simulink library "CTRL_LO_ST1_DFLATLGT"  (R2023b)
settings: Solver=VariableStepAuto  StartTime=0.0  StopTime=10.0  RelTol=1e-3
undefined symbols (not defined in the file): CTRL_LO_ST1_p_DeltaFLgt_N
settings Model: Creator=blatak  LastModifiedBy=blatak

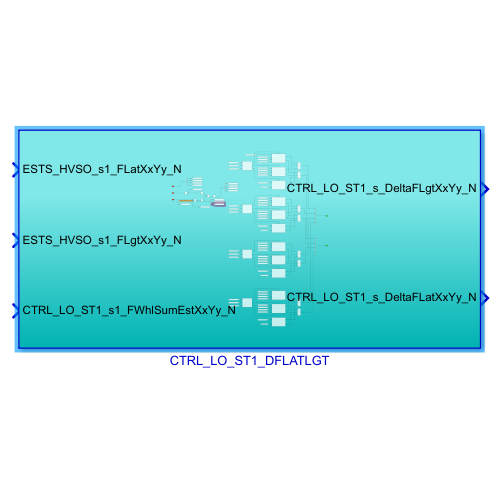
[thumbnail: Simulink's stored preview of the top-level diagram]
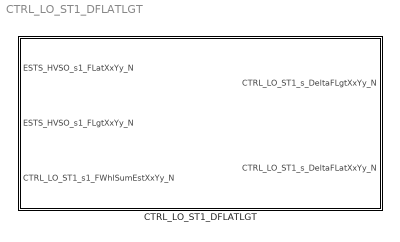
== system CTRL_LO_ST1_DFLATLGT ==
  CTRL_LO_ST1_DFLATLGT : Subsystem

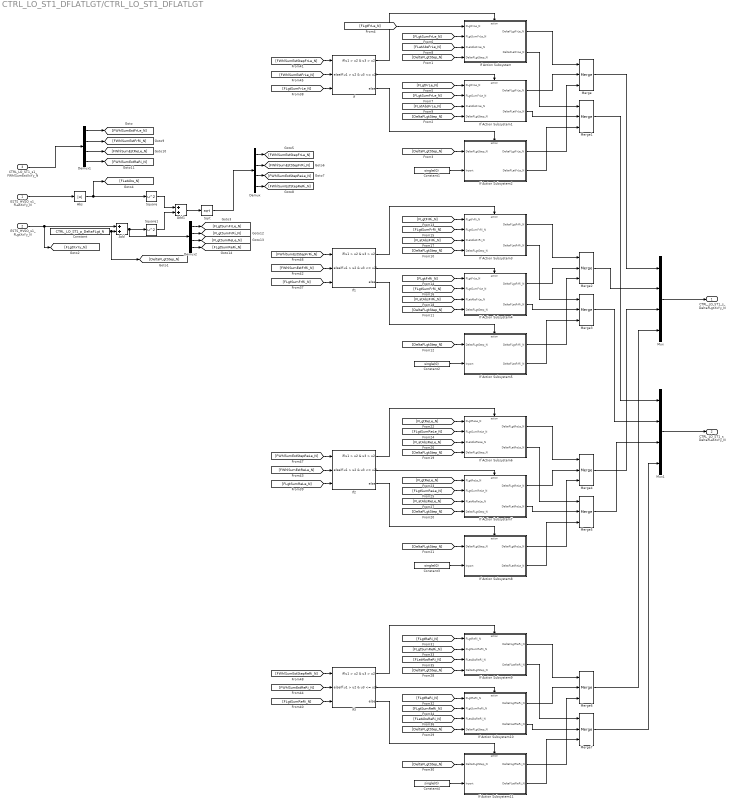
== system CTRL_LO_ST1_DFLATLGT/CTRL_LO_ST1_DFLATLGT ==
  ESTS_HVSO_s1_FLatXxYy_N : Inport
  ESTS_HVSO_s1_FLgtXxYy_N : Inport  Port=2
  CTRL_LO_ST1_s1_FWhlSumEstXxYy_N : Inport  Port=3
  Abs : Abs  SaturateOnIntegerOverflow=off
  Add : Sum
  Add1 : Sum
  Constant : Constant  Value=CTRL_LO_ST1_p_DeltaFLgt_N
  Constant{1..4} (4 alike) : Constant  Value=single(0)
  Demux : Demux
  Demux1 : Demux
  Demux2 : Demux
  If{,1..3} (4 alike) : If  NumInputs=3  IfExpression=u1 > u2 & u3 > u2  ElseIfExpressions=u1 > u2 & u3 <= u2
  If Action Subsystem : Subsystem  TreatAsAtomicUnit=on
  If Action Subsystem1 : Subsystem  TreatAsAtomicUnit=on
  If Action Subsystem10 : Subsystem  AncestorBlock=CTRL_LO_ST1_DFLATLGT/CTRL_LO_ST1_DFLATLGT/If Action Subsystem1  TreatAsAtomicUnit=on
  If Action Subsystem11 : Subsystem  AncestorBlock=CTRL_LO_ST1_DFLATLGT/CTRL_LO_ST1_DFLATLGT/If Action Subsystem2  TreatAsAtomicUnit=on
  If Action Subsystem2 : Subsystem  TreatAsAtomicUnit=on
  If Action Subsystem3 : Subsystem  AncestorBlock=CTRL_LO_ST1_DFLATLGT/CTRL_LO_ST1_DFLATLGT/If Action Subsystem  TreatAsAtomicUnit=on
  If Action Subsystem4 : Subsystem  AncestorBlock=CTRL_LO_ST1_DFLATLGT/CTRL_LO_ST1_DFLATLGT/If Action Subsystem1  TreatAsAtomicUnit=on
  If Action Subsystem5 : Subsystem  AncestorBlock=CTRL_LO_ST1_DFLATLGT/CTRL_LO_ST1_DFLATLGT/If Action Subsystem2  TreatAsAtomicUnit=on
  If Action Subsystem6 : Subsystem  AncestorBlock=CTRL_LO_ST1_DFLATLGT/CTRL_LO_ST1_DFLATLGT/If Action Subsystem  TreatAsAtomicUnit=on
  If Action Subsystem7 : Subsystem  AncestorBlock=CTRL_LO_ST1_DFLATLGT/CTRL_LO_ST1_DFLATLGT/If Action Subsystem1  TreatAsAtomicUnit=on
  If Action Subsystem8 : Subsystem  AncestorBlock=CTRL_LO_ST1_DFLATLGT/CTRL_LO_ST1_DFLATLGT/If Action Subsystem2  TreatAsAtomicUnit=on
  If Action Subsystem9 : Subsystem  AncestorBlock=CTRL_LO_ST1_DFLATLGT/CTRL_LO_ST1_DFLATLGT/If Action Subsystem  TreatAsAtomicUnit=on
  Merge{,1..7} (8 alike) : Merge  Inputs=3
  Mux : Mux
  Mux1 : Mux
  Sqrt : Sqrt
  Square : Math  Operator=square
  Square1 : Math  Operator=square
  CTRL_LO_ST1_s_DeltaFLgtXxYy_N : Outport
  CTRL_LO_ST1_s_DeltaFLatXxYy_N : Outport  Port=2
  wires:
  Abs/1 -> [FLatAbs_N], Square/1
  Add1/1 -> Sqrt/1
  Square/1 -> Add1/1
  Add/1 -> Demux2/1, Square1/1
  If Action Subsystem/1(DeltaFLgtFrLe_N) -> Merge/1
  Merge/1 -> Mux/1
  If/2 -> If Action Subsystem1/Action
  If Action Subsystem2/1(DeltaFLgtFrLe_N) -> Merge/3
  Constant/1 -> [DeltaFLgtStep_N], Add/2
  [FLgtSumFrLe_N] -> If Action Subsystem1/2(FLgtSumFrLe_N)
  If Action Subsystem2/2(DeltaFLatFrLe_N) -> Merge1/3
  [DeltaFLgtStep_N] -> If Action Subsystem2/1(DeltaFLgtStep_N)
  ESTS_HVSO_s1_FLgtXxYy_N/1 -> [FLgtXxYy_N], Add/1
  If Action Subsystem1/2(DeltaFLatFrLe_N) -> Merge1/2
  Sqrt/1 -> Demux/1
  [FLgtSumFrLe_N] -> If Action Subsystem/2(FLgtSumFrLe_N)
  [FLgtFrLe_N] -> If Action Subsystem1/1(FLgtFrLe_N)
  [FLatAbsFrLe_N] -> If Action Subsystem1/3(FLatAbsFrLe_N)
  [DeltaFLgtStep_N] -> If Action Subsystem/4(DeltaFLgtStep_N)
  Square1/1 -> Add1/2
  [DeltaFLgtStep_N] -> If Action Subsystem1/4(DeltaFLgtStep_N)
  Constant1/1 -> If Action Subsystem2/2(Inport)
  ESTS_HVSO_s1_FLatXxYy_N/1 -> Abs/1
  CTRL_LO_ST1_s1_FWhlSumEstXxYy_N/1 -> Demux1/1
  Merge1/1 -> Mux1/1
  [FLgtFrLe_N] -> If Action Subsystem/1(FLgtFrLe_N)
  If/3 -> If Action Subsystem2/Action
  [FLatAbsFrLe_N] -> If Action Subsystem/3(FLatAbsFrLe_N)
  If Action Subsystem1/1(DeltaFLgtFrLe_N) -> Merge/2
  If/1 -> If Action Subsystem/Action
  If Action Subsystem/2(DeltaFLatFrLe_N) -> Merge1/1
  If Action Subsystem5/2(DeltaFLatFrRi_N) -> Merge3/3
  Merge2/1 -> Mux/2
  [FLatAbsFrRi_N] -> If Action Subsystem4/3(FLatAbsFrLe_N)
  If Action Subsystem4/2(DeltaFLatFrRi_N) -> Merge3/2
  [FLgtSumFrRi_N] -> If Action Subsystem3/2(FLgtSumFrRi_N)
  [FLgtFrRi_N] -> If Action Subsystem4/1(FLgtFrLe_N)
  If Action Subsystem3/2(DeltaFLatFrRi_N) -> Merge3/1
  If Action Subsystem4/1(DeltaFLgtFrRi_N) -> Merge2/2
  If1/1 -> If Action Subsystem3/Action
  [DeltaFLgtStep_N] -> If Action Subsystem4/4(DeltaFLgtStep_N)
  [FLgtFrRi_N] -> If Action Subsystem3/1(FLgtFrRi_N)
  Constant2/1 -> If Action Subsystem5/2(Inport)
  [FLatAbsFrRi_N] -> If Action Subsystem3/3(FLatAbsFrRi_N)
  If1/3 -> If Action Subsystem5/Action
  If1/2 -> If Action Subsystem4/Action
  [FLgtSumFrRi_N] -> If Action Subsystem4/2(FLgtSumFrLe_N)
  [DeltaFLgtStep_N] -> If Action Subsystem5/1(DeltaFLgtStep_N)
  [DeltaFLgtStep_N] -> If Action Subsystem3/4(DeltaFLgtStep_N)
  If Action Subsystem3/1(DeltaFLgtFrRi_N) -> Merge2/1
  If Action Subsystem5/1(DeltaFLgtFrRi_N) -> Merge2/3
  Merge3/1 -> Mux1/2
  If Action Subsystem8/2(DeltaFLatReLe_N) -> Merge5/3
  Merge4/1 -> Mux/3
  [FLatAbsReLe_N] -> If Action Subsystem7/3(FLatAbsReLe_N)
  If Action Subsystem7/2(DeltaFLatReLe_N) -> Merge5/2
  [FLgtSumReLe_N] -> If Action Subsystem6/2(FLgtSumReLe_N)
  [FLgtReLe_N] -> If Action Subsystem7/1(FLgtReLe_N)
  If Action Subsystem6/2(DeltaFLatReLe_N) -> Merge5/1
  If Action Subsystem7/1(DeltaFLgtReLe_N) -> Merge4/2
  If2/1 -> If Action Subsystem6/Action
  [DeltaFLgtStep_N] -> If Action Subsystem7/4(DeltaFLgtStep_N)
  [FLgtReLe_N] -> If Action Subsystem6/1(FLgtReLe_N)
  Constant3/1 -> If Action Subsystem8/2(Inport)
  [FLatAbsReLe_N] -> If Action Subsystem6/3(FLatAbsReLe_N)
  If2/3 -> If Action Subsystem8/Action
  If2/2 -> If Action Subsystem7/Action
  [FLgtSumReLe_N] -> If Action Subsystem7/2(FLgtSumReLe_N)
  [DeltaFLgtStep_N] -> If Action Subsystem8/1(DeltaFLgtStep_N)
  [DeltaFLgtStep_N] -> If Action Subsystem6/4(DeltaFLgtStep_N)
  If Action Subsystem6/1(DeltaFLgtReLe_N) -> Merge4/1
  If Action Subsystem8/1(DeltaFLgtReLe_N) -> Merge4/3
  Merge5/1 -> Mux1/3
  If Action Subsystem11/2(DeltaFLatReRi_N) -> Merge7/3
  Merge6/1 -> Mux/4
  [FLatAbsReRi_N] -> If Action Subsystem10/3(FLatAbsReRi_N)
  If Action Subsystem10/2(DeltaFLatReRi_N) -> Merge7/2
  [FLgtSumReRi_N] -> If Action Subsystem9/2(FLgtSumReRi_N)
  [FLgtReRi_N] -> If Action Subsystem10/1(FLgtReRi_N)
  If Action Subsystem9/2(DeltaFLatReRi_N) -> Merge7/1
  If Action Subsystem10/1(DeltaFLgtReRi_N) -> Merge6/2
  If3/1 -> If Action Subsystem9/Action
  [DeltaFLgtStep_N] -> If Action Subsystem10/4(DeltaFLgtStep_N)
  [FLgtReRi_N] -> If Action Subsystem9/1(FLgtReRi_N)
  Constant4/1 -> If Action Subsystem11/2(Inport)
  [FLatAbsReRi_N] -> If Action Subsystem9/3(FLatAbsReRi_N)
  If3/3 -> If Action Subsystem11/Action
  If3/2 -> If Action Subsystem10/Action
  [FLgtSumReRi_N] -> If Action Subsystem10/2(FLgtSumReRi_N)
  [DeltaFLgtStep_N] -> If Action Subsystem11/1(DeltaFLgtStep_N)
  [DeltaFLgtStep_N] -> If Action Subsystem9/4(DeltaFLgtStep_N)
  If Action Subsystem9/1(DeltaFLgtReRi_N) -> Merge6/1
  If Action Subsystem11/1(DeltaFLgtReRi_N) -> Merge6/3
  Merge7/1 -> Mux1/4
  Mux1/1 -> CTRL_LO_ST1_s_DeltaFLatXxYy_N/1
  Mux/1 -> CTRL_LO_ST1_s_DeltaFLgtXxYy_N/1
  [FLgtSumFrRi_N] -> If1/3
  [FLgtSumFrLe_N] -> If/3
  [FLgtSumReLe_N] -> If2/3
  [FLgtSumReRi_N] -> If3/3
  Demux/1 -> [FWhlSumEstStepFrLe_N]
  Demux/2 -> [FWhlSumEstStepFrRi_N]
  Demux/3 -> [FWhlSumEstStepReLe_N]
  Demux/4 -> [FWhlSumEstStepReRi_N]
  [FWhlSumEstStepFrLe_N] -> If/1
  [FWhlSumEstFrRi_N] -> If1/2
  [FWhlSumEstReLe_N] -> If2/2
  [FWhlSumEstReRi_N] -> If3/2
  Demux1/1 -> [FWhlSumEstFrLe_N]
  Demux1/4 -> [FWhlSumEstReRi_N]
  Demux1/3 -> [FWhlSumEstReLe_N]
  Demux1/2 -> [FWhlSumEstFrRi_N]
  [FWhlSumEstFrLe_N] -> If/2
  [FWhlSumEstStepFrRi_N] -> If1/1
  [FWhlSumEstStepReLe_N] -> If2/1
  [FWhlSumEstStepReRi_N] -> If3/1
  Demux2/1 -> [FLgtSumFrLe_N]
  Demux2/2 -> [FLgtSumFrRi_N]
  Demux2/3 -> [FLgtSumReLe_N]
  Demux2/4 -> [FLgtSumReRi_N]

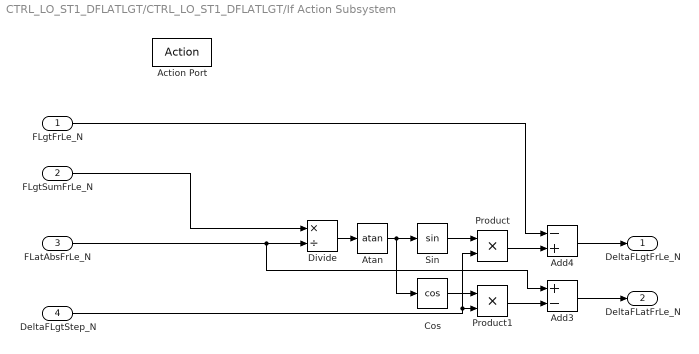
== system CTRL_LO_ST1_DFLATLGT/CTRL_LO_ST1_DFLATLGT/If Action Subsystem ==
  FLgtFrLe_N : Inport
  FLgtSumFrLe_N : Inport  Port=2
  FLatAbsFrLe_N : Inport  Port=3
  DeltaFLgtStep_N : Inport  Port=4
  Action Port : ActionPort  ActionPortLabel=if(u1 > u2 & u3 > u2)
  Add3 : Sum  Inputs=+-
  Add4 : Sum  Inputs=-+
  Atan : Trigonometry  Operator=atan
  Cos : Trigonometry  Operator=cos
  Divide : Product  Inputs=*/
  Product : Product
  Product1 : Product
  Sin : Trigonometry
  DeltaFLgtFrLe_N : Outport
  DeltaFLatFrLe_N : Outport  Port=2
  wires:
  Add4/1 -> DeltaFLgtFrLe_N/1
  Add3/1 -> DeltaFLatFrLe_N/1
  Cos/1 -> Product1/1
  Product/1 -> Add4/2
  Atan/1 -> Cos/1, Sin/1
  Sin/1 -> Product/1
  Divide/1 -> Atan/1
  FLatAbsFrLe_N/1 -> Divide/2, Add3/1
  Product1/1 -> Add3/2
  DeltaFLgtStep_N/1 -> Product/2, Product1/2
  FLgtSumFrLe_N/1 -> Divide/1
  FLgtFrLe_N/1 -> Add4/1

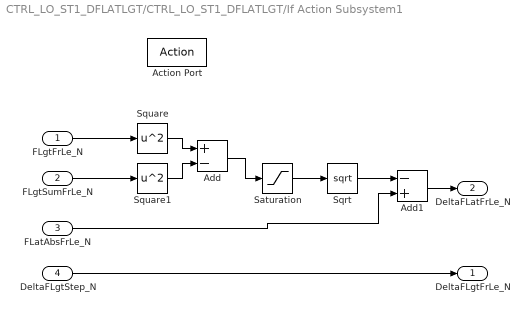
== system CTRL_LO_ST1_DFLATLGT/CTRL_LO_ST1_DFLATLGT/If Action Subsystem1 ==
  FLgtFrLe_N : Inport
  FLgtSumFrLe_N : Inport  Port=2
  FLatAbsFrLe_N : Inport  Port=3
  DeltaFLgtStep_N : Inport  Port=4
  Action Port : ActionPort  ActionPortLabel=elseif(u1 > u2 & u3 <= u2)
  Add : Sum  Inputs=+-
  Add1 : Sum  Inputs=-+
  Saturation : Saturate  UpperLimit=Inf  LowerLimit=0
  Sqrt : Sqrt
  Square : Math  Operator=square
  Square1 : Math  Operator=square
  DeltaFLgtFrLe_N : Outport
  DeltaFLatFrLe_N : Outport  Port=2
  wires:
  Sqrt/1 -> Add1/1
  Add1/1 -> DeltaFLatFrLe_N/1
  DeltaFLgtStep_N/1 -> DeltaFLgtFrLe_N/1
  Square/1 -> Add/1
  FLgtSumFrLe_N/1 -> Square1/1
  FLgtFrLe_N/1 -> Square/1
  FLatAbsFrLe_N/1 -> Add1/2
  Add/1 -> Saturation/1
  Saturation/1 -> Sqrt/1
  Square1/1 -> Add/2

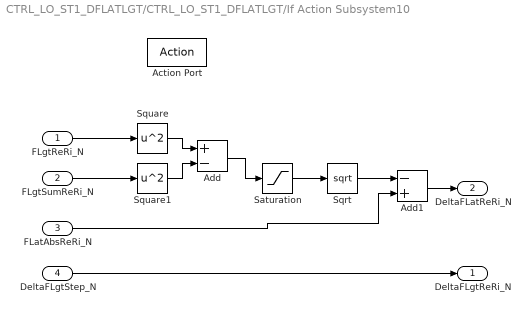
== system CTRL_LO_ST1_DFLATLGT/CTRL_LO_ST1_DFLATLGT/If Action Subsystem10 ==
  FLgtReRi_N : Inport
  FLgtSumReRi_N : Inport  Port=2
  FLatAbsReRi_N : Inport  Port=3
  DeltaFLgtStep_N : Inport  Port=4
  Action Port : ActionPort
  Add : Sum  Inputs=+-
  Add1 : Sum  Inputs=-+
  Saturation : Saturate  UpperLimit=Inf  LowerLimit=0
  Sqrt : Sqrt
  Square : Math  Operator=square
  Square1 : Math  Operator=square
  DeltaFLgtReRi_N : Outport
  DeltaFLatReRi_N : Outport  Port=2
  wires:
  Square1/1 -> Add/2
  Saturation/1 -> Sqrt/1
  Add/1 -> Saturation/1
  FLatAbsReRi_N/1 -> Add1/2
  FLgtReRi_N/1 -> Square/1
  FLgtSumReRi_N/1 -> Square1/1
  Square/1 -> Add/1
  DeltaFLgtStep_N/1 -> DeltaFLgtReRi_N/1
  Add1/1 -> DeltaFLatReRi_N/1
  Sqrt/1 -> Add1/1

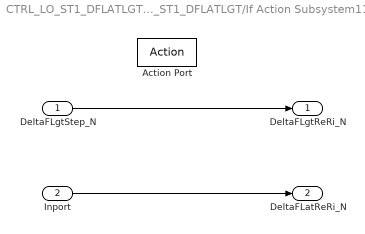
== system CTRL_LO_ST1_DFLATLGT/CTRL_LO_ST1_DFLATLGT/If Action Subsystem11 ==
  DeltaFLgtStep_N : Inport
  Inport : Inport  Port=2
  Action Port : ActionPort
  DeltaFLgtReRi_N : Outport
  DeltaFLatReRi_N : Outport  Port=2
  wires:
  Inport/1 -> DeltaFLatReRi_N/1
  DeltaFLgtStep_N/1 -> DeltaFLgtReRi_N/1

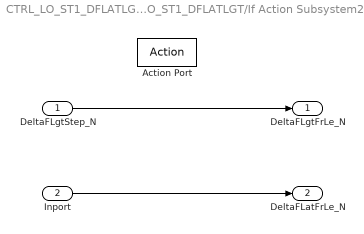
== system CTRL_LO_ST1_DFLATLGT/CTRL_LO_ST1_DFLATLGT/If Action Subsystem2 ==
  DeltaFLgtStep_N : Inport
  Inport : Inport  Port=2
  Action Port : ActionPort  ActionPortLabel=else
  DeltaFLgtFrLe_N : Outport
  DeltaFLatFrLe_N : Outport  Port=2
  wires:
  DeltaFLgtStep_N/1 -> DeltaFLgtFrLe_N/1
  Inport/1 -> DeltaFLatFrLe_N/1

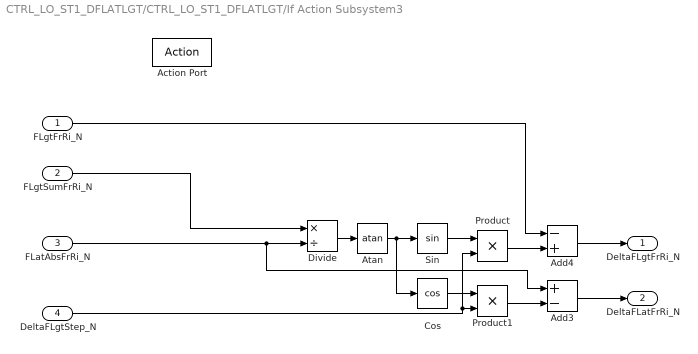
== system CTRL_LO_ST1_DFLATLGT/CTRL_LO_ST1_DFLATLGT/If Action Subsystem3 ==
  FLgtFrRi_N : Inport
  FLgtSumFrRi_N : Inport  Port=2
  FLatAbsFrRi_N : Inport  Port=3
  DeltaFLgtStep_N : Inport  Port=4
  Action Port : ActionPort
  Add3 : Sum  Inputs=+-
  Add4 : Sum  Inputs=-+
  Atan : Trigonometry  Operator=atan
  Cos : Trigonometry  Operator=cos
  Divide : Product  Inputs=*/
  Product : Product
  Product1 : Product
  Sin : Trigonometry
  DeltaFLgtFrRi_N : Outport
  DeltaFLatFrRi_N : Outport  Port=2
  wires:
  FLgtFrRi_N/1 -> Add4/1
  FLgtSumFrRi_N/1 -> Divide/1
  DeltaFLgtStep_N/1 -> Product1/2, Product/2
  Product1/1 -> Add3/2
  FLatAbsFrRi_N/1 -> Add3/1, Divide/2
  Divide/1 -> Atan/1
  Sin/1 -> Product/1
  Atan/1 -> Sin/1, Cos/1
  Product/1 -> Add4/2
  Cos/1 -> Product1/1
  Add3/1 -> DeltaFLatFrRi_N/1
  Add4/1 -> DeltaFLgtFrRi_N/1

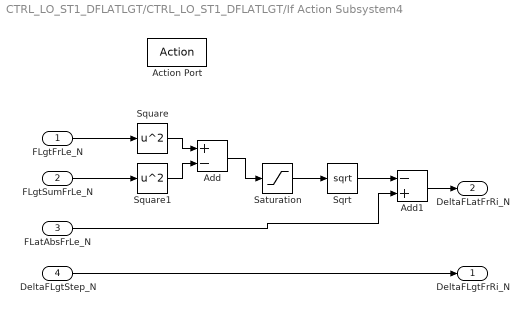
== system CTRL_LO_ST1_DFLATLGT/CTRL_LO_ST1_DFLATLGT/If Action Subsystem4 ==
  FLgtFrLe_N : Inport
  FLgtSumFrLe_N : Inport  Port=2
  FLatAbsFrLe_N : Inport  Port=3
  DeltaFLgtStep_N : Inport  Port=4
  Action Port : ActionPort
  Add : Sum  Inputs=+-
  Add1 : Sum  Inputs=-+
  Saturation : Saturate  UpperLimit=Inf  LowerLimit=0
  Sqrt : Sqrt
  Square : Math  Operator=square
  Square1 : Math  Operator=square
  DeltaFLgtFrRi_N : Outport
  DeltaFLatFrRi_N : Outport  Port=2
  wires:
  Square1/1 -> Add/2
  Saturation/1 -> Sqrt/1
  Add/1 -> Saturation/1
  FLatAbsFrLe_N/1 -> Add1/2
  FLgtFrLe_N/1 -> Square/1
  FLgtSumFrLe_N/1 -> Square1/1
  Square/1 -> Add/1
  DeltaFLgtStep_N/1 -> DeltaFLgtFrRi_N/1
  Add1/1 -> DeltaFLatFrRi_N/1
  Sqrt/1 -> Add1/1

== system CTRL_LO_ST1_DFLATLGT/CTRL_LO_ST1_DFLATLGT/If Action Subsystem5 ==
  DeltaFLgtStep_N : Inport
  Inport : Inport  Port=2
  Action Port : ActionPort
  DeltaFLgtFrRi_N : Outport
  DeltaFLatFrRi_N : Outport  Port=2
  wires:
  Inport/1 -> DeltaFLatFrRi_N/1
  DeltaFLgtStep_N/1 -> DeltaFLgtFrRi_N/1

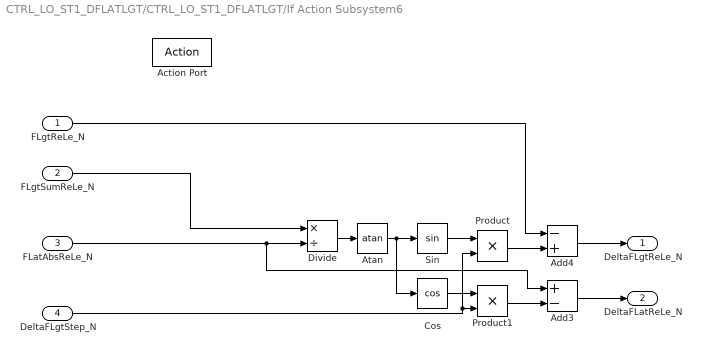
== system CTRL_LO_ST1_DFLATLGT/CTRL_LO_ST1_DFLATLGT/If Action Subsystem6 ==
  FLgtReLe_N : Inport
  FLgtSumReLe_N : Inport  Port=2
  FLatAbsReLe_N : Inport  Port=3
  DeltaFLgtStep_N : Inport  Port=4
  Action Port : ActionPort
  Add3 : Sum  Inputs=+-
  Add4 : Sum  Inputs=-+
  Atan : Trigonometry  Operator=atan
  Cos : Trigonometry  Operator=cos
  Divide : Product  Inputs=*/
  Product : Product
  Product1 : Product
  Sin : Trigonometry
  DeltaFLgtReLe_N : Outport
  DeltaFLatReLe_N : Outport  Port=2
  wires:
  FLgtReLe_N/1 -> Add4/1
  FLgtSumReLe_N/1 -> Divide/1
  DeltaFLgtStep_N/1 -> Product1/2, Product/2
  Product1/1 -> Add3/2
  FLatAbsReLe_N/1 -> Add3/1, Divide/2
  Divide/1 -> Atan/1
  Sin/1 -> Product/1
  Atan/1 -> Sin/1, Cos/1
  Product/1 -> Add4/2
  Cos/1 -> Product1/1
  Add3/1 -> DeltaFLatReLe_N/1
  Add4/1 -> DeltaFLgtReLe_N/1

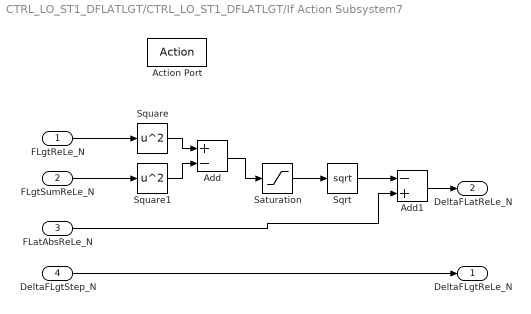
== system CTRL_LO_ST1_DFLATLGT/CTRL_LO_ST1_DFLATLGT/If Action Subsystem7 ==
  FLgtReLe_N : Inport
  FLgtSumReLe_N : Inport  Port=2
  FLatAbsReLe_N : Inport  Port=3
  DeltaFLgtStep_N : Inport  Port=4
  Action Port : ActionPort
  Add : Sum  Inputs=+-
  Add1 : Sum  Inputs=-+
  Saturation : Saturate  UpperLimit=Inf  LowerLimit=0
  Sqrt : Sqrt
  Square : Math  Operator=square
  Square1 : Math  Operator=square
  DeltaFLgtReLe_N : Outport
  DeltaFLatReLe_N : Outport  Port=2
  wires:
  Square1/1 -> Add/2
  Saturation/1 -> Sqrt/1
  Add/1 -> Saturation/1
  FLatAbsReLe_N/1 -> Add1/2
  FLgtReLe_N/1 -> Square/1
  FLgtSumReLe_N/1 -> Square1/1
  Square/1 -> Add/1
  DeltaFLgtStep_N/1 -> DeltaFLgtReLe_N/1
  Add1/1 -> DeltaFLatReLe_N/1
  Sqrt/1 -> Add1/1

== system CTRL_LO_ST1_DFLATLGT/CTRL_LO_ST1_DFLATLGT/If Action Subsystem8 ==
  DeltaFLgtStep_N : Inport
  Inport : Inport  Port=2
  Action Port : ActionPort
  DeltaFLgtReLe_N : Outport
  DeltaFLatReLe_N : Outport  Port=2
  wires:
  Inport/1 -> DeltaFLatReLe_N/1
  DeltaFLgtStep_N/1 -> DeltaFLgtReLe_N/1

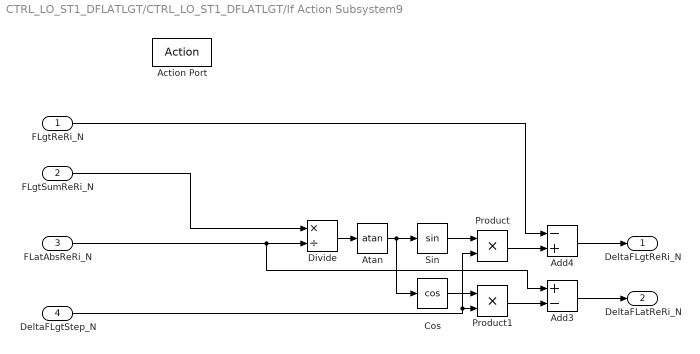
== system CTRL_LO_ST1_DFLATLGT/CTRL_LO_ST1_DFLATLGT/If Action Subsystem9 ==
  FLgtReRi_N : Inport
  FLgtSumReRi_N : Inport  Port=2
  FLatAbsReRi_N : Inport  Port=3
  DeltaFLgtStep_N : Inport  Port=4
  Action Port : ActionPort
  Add3 : Sum  Inputs=+-
  Add4 : Sum  Inputs=-+
  Atan : Trigonometry  Operator=atan
  Cos : Trigonometry  Operator=cos
  Divide : Product  Inputs=*/
  Product : Product
  Product1 : Product
  Sin : Trigonometry
  DeltaFLgtReRi_N : Outport
  DeltaFLatReRi_N : Outport  Port=2
  wires:
  FLgtReRi_N/1 -> Add4/1
  FLgtSumReRi_N/1 -> Divide/1
  DeltaFLgtStep_N/1 -> Product1/2, Product/2
  Product1/1 -> Add3/2
  FLatAbsReRi_N/1 -> Add3/1, Divide/2
  Divide/1 -> Atan/1
  Sin/1 -> Product/1
  Atan/1 -> Sin/1, Cos/1
  Product/1 -> Add4/2
  Cos/1 -> Product1/1
  Add3/1 -> DeltaFLatReRi_N/1
  Add4/1 -> DeltaFLgtReRi_N/1
